simulink model "heli_close_edit"  (R2021a)
settings: Solver=VariableStepAuto  StartTime=0.0  StopTime=10.0  RelTol=1e-3
values from neighbouring files (symbols this model uses):
  A = [-0.4 0 -0.01 ... (first row only)    [heli.m]
  B = [6.3 0 9.8]'    [heli.m]
  K = [eval(KSO.K1) eval(KSO.K2) eval(KSO.K3)]    [heli.m]
settings Model: Creator=McQueen_Zero  LastModifiedBy=McQueen_Zero

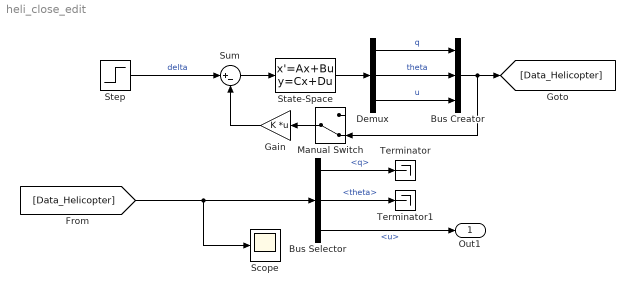
== system heli_close_edit ==
  Bus Creator : BusCreator  Inputs=3
  Bus Selector : BusSelector  OutputSignals=q,theta,u
  Demux : Demux  Outputs=3
  Gain : Gain  Gain=K  Multiplication=Matrix(K*u)
  Manual Switch : ManualSwitch  CurrentSetting=0
  Scope : Scope
  State-Space : StateSpace  A=A  B=B  C=eye(3)  D=[0 0 0]'  InitialCondition=0
  Step : Step  SampleTime=0
  Sum : Sum  Inputs=|+-
  Terminator : Terminator
  Terminator1 : Terminator
  Out1 : Outport
  wires:
  State-Space/1 -> Demux/1
  Demux/1 -> Bus Creator/1  "q"
  Demux/2 -> Bus Creator/2  "theta"
  Demux/3 -> Bus Creator/3  "u"
  Bus Creator/1 -> Manual Switch/2, [Data_Helicopter]
  [Data_Helicopter] -> Scope/1, Bus Selector/1
  Step/1 -> Sum/1  "delta"
  Bus Selector/3 -> Out1/1  "<u>"
  Bus Selector/1 -> Terminator/1  "<q>"
  Bus Selector/2 -> Terminator1/1  "<theta>"
  Sum/1 -> State-Space/1
  Manual Switch/1 -> Gain/1
  Gain/1 -> Sum/2
